simulink model "VTOLAutopilotController"  (R2025a)
settings: configuration reference "VTOLConfiguration" (kept outside this file)
undefined symbols (not defined in the file): Back_Transition_Rate, const, control, controlParams, ControlSampleTime, CriticalTiltAngle, DiscIntNeverNeededParam, dspblkCoreblockFVToolHelper, Fading_time, flightState, FSState, FWControlParams, FWTrimSpeed, gcbh, HoverMission, ReferenceFilterDen, ReferenceFilterNum, tilt_max, tiltIni, TransitioncontrolGains, uavParam, uavParams, VTOLcontrolGains, w_trim, WindDownRate
libraries: simulink x43, slpidlib x35, uavalgslib x7, simulink_extras x1
(part 5 of 8)

== system VTOLAutopilotController/Low level controller/Fixed Wing Controller/Fixed Wing Controller Module/Fixed Wing Controller Tuning/Airspeed-Altitude Controller ==
  note: Airspeed and altitude are controlled independently
      | by ignoring their coupled dynamics.
  Airspeed SP : Inport
  Altitude SP : Inport  Port=2
  Climb Rate SP : Inport  Port=3
  Airspeed : Inport  Port=4
  xyz : Inport  Port=5
  vxyz : Inport  Port=6
  Enable : EnablePort  ShowOutputPort=on
  Airspeed Controller : slpidlib/PID Controller  Controller=PID  Form=Parallel  TimeDomain=Discrete-time  UseExternalTs=off  SampleTime=ControlSampleTime  IntegratorMethod=Trapezoidal  FilterMethod=Forward Euler  ControllerParametersSource=internal  P=40.1166410885074  I=21.6851560041072  UseKiTs=off  D=2.18528545905044  UseExternalDerivativeSource=off  N=172.44752694034  UseFilter=on  TunerSelectOption=Transfer Function Based (PID Tuner App)  InitialConditionSource=internal  InitialConditionForIntegrator=0  InitialConditionForFilter=0  DifferentiatorICPrevScaledInput=0  ExternalReset=none  TrackingMode=off  Kt=1  LimitOutput=off  SatLimitsSource=internal  UpperSaturationLimit=Inf  LowerSaturationLimit=0  LinearizeAsGain=on  AntiWindupMode=clamping  Kb=1  LimitIntegrator=off  UpperIntegratorSaturationLimit=inf  LowerIntegratorSaturationLimit=-inf  POutMin=[]  POutMax=[]  IOutMin=[]  IOutMax=[]  DOutMin=[]  DOutMax=[]  NOutMin=[]  NOutMax=[]  SumOutMin=[]  SumOutMax=[]  SaturationOutMin=[]  SaturationOutMax=[]  PParamMin=[]  PParamMax=[]  IParamMin=[]  IParamMax=[]  DParamMin=[]  DParamMax=[]  NParamMin=[]  NParamMax=[]  KbParamMin=[]  KbParamMax=[]  KtParamMin=[]  KtParamMax=[]  KbOutMin=[]  KbOutMax=[]  KtOutMin=[]  KtOutMax=[]  IntegratorOutMin=[]  IntegratorOutMax=[]  FilterOutMin=[]  FilterOutMax=[]  SumI1OutMin=[]  SumI1OutMax=[]  SumI2OutMin=[]  SumI2OutMax=[]  SumI3OutMin=[]  SumI3OutMax=[]  SumI4OutMin=[]  SumI4OutMax=[]  SumDOutMin=[]  SumDOutMax=[]  DifferentiatorOutMin=[]  DifferentiatorOutMax=[]  FilterDiffOutCoefMin=[]  FilterDiffOutCoefMax=[]  ReciprocalOutMin=[]  ReciprocalOutMax=[]  SumDenOutMin=[]  SumDenOutMax=[]  SumNumOutMin=[]  SumNumOutMax=[]  DivideOutMin=[]  DivideOutMax=[]  UdiffTsProdOutMin=[]  UdiffTsProdOutMax=[]  NTsProdOutMin=[]  NTsProdOutMax=[]  UintegralTsProdOutMin=[]  UintegralTsProdOutMax=[]  UngainTsProdOutMin=[]  UngainTsProdOutMax=[]  ClampingZeroOutDataTypeStr=Inherit: Inherit via back propagation  ClampingZeroOutMin=[]  ClampingZeroOutMax=[]  FilterDenConstantOutDataTypeStr=Inherit: Inherit via back propagation  FilterDenConstantOutMin=[]  FilterDenConstantOutMax=[]  PCopyOutDataTypeStr=Inherit: Inherit via back propagation  PCopyOutMin=[]  PCopyOutMax=[]  NCopyOutDataTypeStr=Inherit: Inherit via back propagation  NCopyOutMin=[]  NCopyOutMax=[]  IntegratorContinuousStateAttributes=''  IntegratorStateMustResolveToSignalObject=off  IntegratorRTWStateStorageClass=Auto  FilterContinuousStateAttributes=''  FilterStateMustResolveToSignalObject=off  FilterRTWStateStorageClass=Auto  ParallelPVariant=InternalParameters  IdealPVariant=Disabled  IVariant=InternalParameters  DVariant=InternalParameters  IntegratorVariant=Discrete  SatVariant=Disabled  AWVariant=Passthrough  PCopyVariant=Disabled  TRVariant=Disabled  FdbkBlocksVariant=Forward  IdealPFdbkVariant=Disabled  SatFdbkVariant=Disabled  DerivativeFilterVariant=ForwardEulerFilter  NVariant=InternalParameters  NCopyVariant=Disabled  FilterICVariant=InternalICsFilter  IntegratorICVariant=InternalICs  ExternalResetVariant=Disabled  TRSumVariant=Passthrough  SumFdbkVariant=Disabled  SumVariant=Sum_PID  TsampFilterVariant=InternalTs  TsampNgainVariant=Passthrough  TsampIntegralVariant=Disabled_SignalSpec  ExternalSaturationOutDataTypeStr=Inherit: Same as second input  DerivativeSourceVariant=ErrorSignal  PreIntVariant=InternalPreInt
  Altitude Controller : Subsystem
  Climb Rate SP Switch : Switch  Criteria=u2 > Threshold  SaturateOnIntegerOverflow=off  InputSameDT=off
  Climb Rate SP from Guidance : Subsystem  TreatAsAtomicUnit=on
  Compare To Constant : simulink/Logic and Bit Operations/Compare To Constant  relop===  const=uint8(1)  OutDataTypeStr=boolean
  Compare To Constant1 : simulink/Logic and Bit Operations/Compare To Constant  relop===  const=uint8(2)  OutDataTypeStr=boolean
  Pitch SP Controller : Subsystem
  Sum1 : Sum  Inputs=|+-
  Pitch SP : Outport
  Throttle : Outport  Port=2
  wires:
  Airspeed SP/1 -> Sum1/1
  Sum1/1 -> Airspeed Controller/1
  Airspeed/1 -> Sum1/2
  Airspeed Controller/1 -> Throttle/1
  Altitude SP/1 -> Altitude Controller/1(Alt SP)
  xyz/1 -> Altitude Controller/2(xyz)
  vxyz/1 -> Pitch SP Controller/2(vxyz)
  Pitch SP Controller/1(Pitch SP) -> Pitch SP/1
  Enable/1 -> Compare To Constant1/1, Compare To Constant/1
  Compare To Constant/1 -> Climb Rate SP Switch/2, Altitude Controller/Enable
  Compare To Constant1/1 -> Climb Rate SP from Guidance/Enable
  Altitude Controller/1(Climb Rate SP) -> Climb Rate SP Switch/1
  Climb Rate SP from Guidance/1(Out1) -> Climb Rate SP Switch/3
  Climb Rate SP Switch/1 -> Pitch SP Controller/1(Climb Rate SP)
  Climb Rate SP/1 -> Climb Rate SP from Guidance/1(Climb Rate SP)

== system VTOLAutopilotController/Low level controller/Fixed Wing Controller/Fixed Wing Controller Module/Fixed Wing Controller Tuning/Attitude Controller ==
  YPR SP : Inport
  ypr : Inport  Port=2
  Ang Rate : Inport  Port=3
  Airspeed : Inport  Port=4
  Enable : EnablePort  ShowOutputPort=on
  AER Switch : Switch  Criteria=u2 > Threshold  SaturateOnIntegerOverflow=off  InputSameDT=off
  Compare To Constant : simulink/Logic and Bit Operations/Compare To Constant  relop===  const=uint8(1)  OutDataTypeStr=boolean
  Compare To Constant1 : simulink/Logic and Bit Operations/Compare To Constant  relop===  const=uint8(2)  OutDataTypeStr=boolean
  Demux1 : Demux  Outputs=3
  Pitch Roll Controller : Subsystem
  Rudder Heading Controller : Subsystem
  AER : Outport
  wires:
  ypr/1 -> Rudder Heading Controller/2(YPR), Pitch Roll Controller/3(YPR)
  YPR SP/1 -> Demux1/1
  Enable/1 -> Compare To Constant1/1, Compare To Constant/1
  AER Switch/1 -> AER/1
  Compare To Constant/1 -> AER Switch/2, Pitch Roll Controller/Enable
  Pitch Roll Controller/1(AER) -> AER Switch/1
  Rudder Heading Controller/1(AER) -> AER Switch/3
  Demux1/1 -> Rudder Heading Controller/1(Yaw SP)
  Demux1/2 -> Pitch Roll Controller/1(Pitch SP)
  Demux1/3 -> Pitch Roll Controller/2(Roll SP)
  Ang Rate/1 -> Rudder Heading Controller/3(Ang Rate), Pitch Roll Controller/4(Ang Rate)
  Compare To Constant1/1 -> Rudder Heading Controller/Enable
  Airspeed/1 -> Pitch Roll Controller/5(Airspeed)

== system VTOLAutopilotController/Low level controller/Fixed Wing Controller/Fixed Wing Controller Module/Fixed Wing Controller Tuning/Lateral Guidance Logic ==
  note: S. Park, J. Deyst, and J. P. How, "A New Nonlinear Guidance Logic for Trajectory Tracking," Proceedings of the AIAA Guidance, Navigation and Control Conference, Aug 2004. AIAA-2004-4900.
  Course SP : Inport
  L1 Distance : Inport  Port=2
  course : Inport  Port=3
  gndspeed : Inport  Port=4
  Enable : EnablePort
  MATLAB Function : MATLAB Function  TreatAsAtomicUnit=on  SystemSampleTime=ControlSampleTime
  Terminator : Terminator
  Roll SP : Outport
  wires:
  Course SP/1 -> MATLAB Function/1(courseSP)
  course/1 -> MATLAB Function/2(course)
  MATLAB Function/2(rollSP) -> Roll SP/1
  MATLAB Function/1(lacc) -> Terminator/1
  gndspeed/1 -> MATLAB Function/3(groundSpeed)
  L1 Distance/1 -> MATLAB Function/4(L1)

== system VTOLAutopilotController/Low level controller/Fixed Wing Controller/Fixed Wing Controller Module/Fixed Wing Controller Tuning/Pitch, Airspeed SP from Controller ==
  Pitch SP In : Inport
  Airspeed SP : Inport  Port=2
  Airspeed : Inport  Port=3
  Enable : EnablePort
  Airspeed Controller : slpidlib/PID Controller  Controller=PID  Form=Parallel  TimeDomain=Discrete-time  UseExternalTs=off  SampleTime=ControlSampleTime  IntegratorMethod=Trapezoidal  FilterMethod=Forward Euler  ControllerParametersSource=internal  P=FWControlParams.P_AIRSPD  I=FWControlParams.I_AIRSPD  UseKiTs=off  D=FWControlParams.D_AIRSPD  UseExternalDerivativeSource=off  N=FWControlParams.N_AIRSPD  UseFilter=on  TunerSelectOption=Transfer Function Based (PID Tuner App)  InitialConditionSource=internal  InitialConditionForIntegrator=0  InitialConditionForFilter=0  DifferentiatorICPrevScaledInput=0  ExternalReset=none  TrackingMode=off  Kt=1  LimitOutput=off  SatLimitsSource=internal  UpperSaturationLimit=Inf  LowerSaturationLimit=0  LinearizeAsGain=on  AntiWindupMode=clamping  Kb=1  LimitIntegrator=off  UpperIntegratorSaturationLimit=inf  LowerIntegratorSaturationLimit=-inf  POutMin=[]  POutMax=[]  IOutMin=[]  IOutMax=[]  DOutMin=[]  DOutMax=[]  NOutMin=[]  NOutMax=[]  SumOutMin=[]  SumOutMax=[]  SaturationOutMin=[]  SaturationOutMax=[]  PParamMin=[]  PParamMax=[]  IParamMin=[]  IParamMax=[]  DParamMin=[]  DParamMax=[]  NParamMin=[]  NParamMax=[]  KbParamMin=[]  KbParamMax=[]  KtParamMin=[]  KtParamMax=[]  KbOutMin=[]  KbOutMax=[]  KtOutMin=[]  KtOutMax=[]  IntegratorOutMin=[]  IntegratorOutMax=[]  FilterOutMin=[]  FilterOutMax=[]  SumI1OutMin=[]  SumI1OutMax=[]  SumI2OutMin=[]  SumI2OutMax=[]  SumI3OutMin=[]  SumI3OutMax=[]  SumI4OutMin=[]  SumI4OutMax=[]  SumDOutMin=[]  SumDOutMax=[]  DifferentiatorOutMin=[]  DifferentiatorOutMax=[]  FilterDiffOutCoefMin=[]  FilterDiffOutCoefMax=[]  ReciprocalOutMin=[]  ReciprocalOutMax=[]  SumDenOutMin=[]  SumDenOutMax=[]  SumNumOutMin=[]  SumNumOutMax=[]  DivideOutMin=[]  DivideOutMax=[]  UdiffTsProdOutMin=[]  UdiffTsProdOutMax=[]  NTsProdOutMin=[]  NTsProdOutMax=[]  UintegralTsProdOutMin=[]  UintegralTsProdOutMax=[]  UngainTsProdOutMin=[]  UngainTsProdOutMax=[]  ClampingZeroOutDataTypeStr=Inherit: Inherit via back propagation  ClampingZeroOutMin=[]  ClampingZeroOutMax=[]  FilterDenConstantOutDataTypeStr=Inherit: Inherit via back propagation  FilterDenConstantOutMin=[]  FilterDenConstantOutMax=[]  PCopyOutDataTypeStr=Inherit: Inherit via back propagation  PCopyOutMin=[]  PCopyOutMax=[]  NCopyOutDataTypeStr=Inherit: Inherit via back propagation  NCopyOutMin=[]  NCopyOutMax=[]  IntegratorContinuousStateAttributes=''  IntegratorStateMustResolveToSignalObject=off  IntegratorRTWStateStorageClass=Auto  FilterContinuousStateAttributes=''  FilterStateMustResolveToSignalObject=off  FilterRTWStateStorageClass=Auto  ParallelPVariant=InternalParameters  IdealPVariant=Disabled  IVariant=InternalParameters  DVariant=InternalParameters  IntegratorVariant=Discrete  SatVariant=Disabled  AWVariant=Passthrough  PCopyVariant=Disabled  TRVariant=Disabled  FdbkBlocksVariant=Forward  IdealPFdbkVariant=Disabled  SatFdbkVariant=Disabled  DerivativeFilterVariant=ForwardEulerFilter  NVariant=InternalParameters  NCopyVariant=Disabled  FilterICVariant=InternalICsFilter  IntegratorICVariant=InternalICs  ExternalResetVariant=Disabled  TRSumVariant=Passthrough  SumFdbkVariant=Disabled  SumVariant=Sum_PID  TsampFilterVariant=InternalTs  TsampNgainVariant=Passthrough  TsampIntegralVariant=Disabled_SignalSpec  ExternalSaturationOutDataTypeStr=Inherit: Same as second input  DerivativeSourceVariant=ErrorSignal  PreIntVariant=InternalPreInt
  IC : InitialCondition  Value=0
  Sum1 : Sum  Inputs=|+-
  Pitch SP : Outport
  Throttle : Outport  Port=2
  wires:
  IC/1 -> Pitch SP/1
  Pitch SP In/1 -> IC/1
  Airspeed SP/1 -> Sum1/1
  Sum1/1 -> Airspeed Controller/1
  Airspeed/1 -> Sum1/2
  Airspeed Controller/1 -> Throttle/1

== system VTOLAutopilotController/Low level controller/Fixed Wing Controller/Fixed Wing Controller Module/Fixed Wing Controller Tuning/Roll SP from Path Manager ==
  In1 : Inport
  Enable : EnablePort
  IC : InitialCondition  Value=0
  Out1 : Outport
  wires:
  In1/1 -> IC/1
  IC/1 -> Out1/1

== system VTOLAutopilotController/Low level controller/Fixed Wing Controller/Fixed Wing Controller Module/Fixed Wing Controller Tuning/Subsystem2 ==
  Euler : Inport
  pqr : Inport  Port=2
  Demux : Demux  Outputs=3
  Display : Display
  MATLAB Function : MATLAB Function  TreatAsAtomicUnit=on
  Matrix Multiply : Product  Multiplication=Matrix(*)
  Terminator : Terminator
  Euler Rate : Outport
  wires:
  Demux/1 -> MATLAB Function/1(phi)
  Demux/2 -> MATLAB Function/2(theta)
  MATLAB Function/1(y) -> Matrix Multiply/1
  pqr/1 -> Matrix Multiply/2
  Euler/1 -> Demux/1
  Demux/3 -> Terminator/1
  Matrix Multiply/1 -> Display/1, Euler Rate/1

== system VTOLAutopilotController/Low level controller/Multicopter Controller/Attitude & Altitude controller/Altitude Control/Alt signal condition ==
  Z_in : Inport
  Constant : Constant  Value=0  SampleTime=-1
  Gain : Gain  Gain=-1
  Gain1 : Gain  Gain=-1
  Saturation Dynamic : simulink/Discontinuities/Saturation Dynamic  OutMin=[]  OutMax=[]  OutDataTypeStr=Inherit: Same as second input  OutDataType=fixdt(1, 16)  OutScaling=2^-10  DoSatur=off
  Z_out : Outport
  wires:
  Z_in/1 -> Gain/1
  Gain/1 -> Saturation Dynamic/1, Saturation Dynamic/2
  Constant/1 -> Saturation Dynamic/3
  Saturation Dynamic/1 -> Gain1/1
  Gain1/1 -> Z_out/1

== system VTOLAutopilotController/Low level controller/Multicopter Controller/Attitude & Altitude controller/Altitude Control/Triggered Subsystem ==
  AltHold : Inport
  Trigger : TriggerPort  VariantControl=(inherit)
  Reference : Outport
  wires:
  AltHold/1 -> Reference/1

== system VTOLAutopilotController/Low level controller/Multicopter Controller/Horizontal Position Control/XY Controller/Forward position ==
  e_y : Inport
  e_x : Inport  Port=2
  sin : Inport  Port=3
  cos : Inport  Port=4
  Add : Sum
  Product : Product
  Product1 : Product
  ef : Outport
  wires:
  Add/1 -> ef/1
  Product1/1 -> Add/2
  Product/1 -> Add/1
  e_x/1 -> Product/2
  e_y/1 -> Product1/1
  sin/1 -> Product1/2
  cos/1 -> Product/1

== system VTOLAutopilotController/Low level controller/Multicopter Controller/Horizontal Position Control/XY Controller/Forward velocity ==
  vy : Inport
  vx : Inport  Port=2
  sin : Inport  Port=3
  cos : Inport  Port=4
  Add : Sum
  Product : Product
  Product1 : Product
  ef : Outport
  wires:
  cos/1 -> Product/1
  sin/1 -> Product1/2
  vy/1 -> Product1/1
  vx/1 -> Product/2
  Product/1 -> Add/1
  Product1/1 -> Add/2
  Add/1 -> ef/1

== system VTOLAutopilotController/Low level controller/Multicopter Controller/Horizontal Position Control/XY Controller/Lateral position ==
  e_y : Inport
  e_x : Inport  Port=2
  sin : Inport  Port=3
  cos : Inport  Port=4
  Add : Sum
  Gain : Gain  Gain=-1
  Product : Product
  Product1 : Product
  el : Outport
  wires:
  e_y/1 -> Product1/1
  e_x/1 -> Product/2
  sin/1 -> Product/1
  cos/1 -> Product1/2
  Product/1 -> Gain/1
  Product1/1 -> Add/2
  Add/1 -> el/1
  Gain/1 -> Add/1

== system VTOLAutopilotController/Low level controller/Multicopter Controller/Horizontal Position Control/XY Controller/Lateral velocity ==
  vy : Inport
  vx : Inport  Port=2
  sin : Inport  Port=3
  cos : Inport  Port=4
  Add : Sum
  Gain : Gain  Gain=-1
  Product : Product
  Product1 : Product
  el : Outport
  wires:
  Gain/1 -> Add/1
  Add/1 -> el/1
  Product1/1 -> Add/2
  Product/1 -> Gain/1
  cos/1 -> Product1/2
  sin/1 -> Product/1
  vx/1 -> Product/2
  vy/1 -> Product1/1

== system VTOLAutopilotController/Low level controller/Scheduler/FixedWingScheduler/Switch Case Action Subsystem3/Signal_Fader_OnOff1 ==
  SW : Inport
  Input_On : Inport  Port=2
  Input_Off : Inport  Port=3
  Fading_Time : Inport  Port=4
  Compare To Constant : simulink/Logic and Bit Operations/Compare To Constant  relop===  const=0  OutDataTypeStr=boolean
  Fader_Off : Subsystem
  Fader_On : Subsystem
  Product : Product
  Product1 : Product
  Sum{,1..3} (4 alike) : Sum  Inputs=+-
  Switch : Switch  Criteria=u2 > Threshold  SaturateOnIntegerOverflow=off  InputSameDT=off
  Switch1 : Switch  Criteria=u2 > Threshold  SaturateOnIntegerOverflow=off  InputSameDT=off
  Switch2 : Switch  Criteria=u2 > Threshold  SaturateOnIntegerOverflow=off  InputSameDT=off
  Unit Delay : UnitDelay  SampleTime=-1  HasFrameUpgradeWarning=on
  Unit Delay1 : UnitDelay  SampleTime=-1  HasFrameUpgradeWarning=on
  Unit Delay2 : UnitDelay  SampleTime=-1  HasFrameUpgradeWarning=on
  Out : Outport
  wires:
  SW/1 -> [Engage]
  Fading_Time/1 -> [Fade_Time]
  [Engage] -> Fader_On/1(SW)
  [Fade_Time] -> Fader_On/2(Fader_Time)
  [Engage] -> Compare To Constant/1
  Compare To Constant/1 -> Fader_Off/1(SW)
  [Fade_Time] -> Fader_Off/2(Fader_Time)
  Input_On/1 -> [On_Input]
  Input_Off/1 -> [Off_Input]
  Unit Delay/1 -> [Out_Capture]
  Switch/1 -> Unit Delay/1, Out/1
  [On_Input] -> Sum/1
  Sum/1 -> Switch/1
  [On_Input] -> Sum1/1
  [Out_Capture] -> Sum1/2
  Sum1/1 -> Switch1/3
  Switch1/1 -> Unit Delay1/1, Product/1
  Unit Delay1/1 -> Switch1/1
  [Engage] -> Switch1/2
  Product/1 -> Sum/2
  Fader_On/1(On) -> Product/2
  [Engage] -> Switch/2
  Sum2/1 -> Switch/3
  Product1/1 -> Sum2/2
  [Off_Input] -> Sum2/1
  [Off_Input] -> Sum3/1
  [Engage] -> Switch2/2
  [Out_Capture] -> Sum3/2
  Sum3/1 -> Switch2/1
  Switch2/1 -> Unit Delay2/1, Product1/2
  Unit Delay2/1 -> Switch2/3
  Fader_Off/1(On) -> Product1/1

== system VTOLAutopilotController/Low level controller/Scheduler/Subsystem/Switch Case Action Subsystem3/Signal_Fader_OnOff ==
  SW : Inport
  Input_On : Inport  Port=2
  Input_Off : Inport  Port=3
  Fading_Time : Inport  Port=4
  Compare To Constant : simulink/Logic and Bit Operations/Compare To Constant  relop===  const=0  OutDataTypeStr=boolean
  Fader_Off : Subsystem
  Fader_On : Subsystem
  Product : Product
  Product1 : Product
  Sum{,1..3} (4 alike) : Sum  Inputs=+-
  Switch : Switch  Criteria=u2 > Threshold  SaturateOnIntegerOverflow=off  InputSameDT=off
  Switch1 : Switch  Criteria=u2 > Threshold  SaturateOnIntegerOverflow=off  InputSameDT=off
  Switch2 : Switch  Criteria=u2 > Threshold  SaturateOnIntegerOverflow=off  InputSameDT=off
  Unit Delay : UnitDelay  SampleTime=-1  HasFrameUpgradeWarning=on
  Unit Delay1 : UnitDelay  SampleTime=-1  HasFrameUpgradeWarning=on
  Unit Delay2 : UnitDelay  SampleTime=-1  HasFrameUpgradeWarning=on
  Out : Outport
  wires:
  SW/1 -> [Engage]
  Fading_Time/1 -> [Fade_Time]
  [Engage] -> Fader_On/1(SW)
  [Fade_Time] -> Fader_On/2(Fader_Time)
  [Engage] -> Compare To Constant/1
  Compare To Constant/1 -> Fader_Off/1(SW)
  [Fade_Time] -> Fader_Off/2(Fader_Time)
  Input_On/1 -> [On_Input]
  Input_Off/1 -> [Off_Input]
  Unit Delay/1 -> [Out_Capture]
  Switch/1 -> Unit Delay/1, Out/1
  [On_Input] -> Sum/1
  Sum/1 -> Switch/1
  [On_Input] -> Sum1/1
  [Out_Capture] -> Sum1/2
  Sum1/1 -> Switch1/3
  Switch1/1 -> Unit Delay1/1, Product/1
  Unit Delay1/1 -> Switch1/1
  [Engage] -> Switch1/2
  Product/1 -> Sum/2
  Fader_On/1(On) -> Product/2
  [Engage] -> Switch/2
  Sum2/1 -> Switch/3
  Product1/1 -> Sum2/2
  [Off_Input] -> Sum2/1
  [Off_Input] -> Sum3/1
  [Engage] -> Switch2/2
  [Out_Capture] -> Sum3/2
  Sum3/1 -> Switch2/1
  Switch2/1 -> Unit Delay2/1, Product1/2
  Unit Delay2/1 -> Switch2/3
  Fader_Off/1(On) -> Product1/1

== system VTOLAutopilotController/Low level controller/Scheduler/Subsystem/Switch Case Action Subsystem3/Signal_Fader_OnOff1 ==
  SW : Inport
  Input_On : Inport  Port=2
  Input_Off : Inport  Port=3
  Fading_Time : Inport  Port=4
  Compare To Constant : simulink/Logic and Bit Operations/Compare To Constant  relop===  const=0  OutDataTypeStr=boolean
  Fader_Off : Subsystem
  Fader_On : Subsystem
  Product : Product
  Product1 : Product
  Sum{,1..3} (4 alike) : Sum  Inputs=+-
  Switch : Switch  Criteria=u2 > Threshold  SaturateOnIntegerOverflow=off  InputSameDT=off
  Switch1 : Switch  Criteria=u2 > Threshold  SaturateOnIntegerOverflow=off  InputSameDT=off
  Switch2 : Switch  Criteria=u2 > Threshold  SaturateOnIntegerOverflow=off  InputSameDT=off
  Unit Delay : UnitDelay  SampleTime=-1  HasFrameUpgradeWarning=on
  Unit Delay1 : UnitDelay  SampleTime=-1  HasFrameUpgradeWarning=on
  Unit Delay2 : UnitDelay  SampleTime=-1  HasFrameUpgradeWarning=on
  Out : Outport
  wires:
  SW/1 -> [Engage]
  Fading_Time/1 -> [Fade_Time]
  [Engage] -> Fader_On/1(SW)
  [Fade_Time] -> Fader_On/2(Fader_Time)
  [Engage] -> Compare To Constant/1
  Compare To Constant/1 -> Fader_Off/1(SW)
  [Fade_Time] -> Fader_Off/2(Fader_Time)
  Input_On/1 -> [On_Input]
  Input_Off/1 -> [Off_Input]
  Unit Delay/1 -> [Out_Capture]
  Switch/1 -> Unit Delay/1, Out/1
  [On_Input] -> Sum/1
  Sum/1 -> Switch/1
  [On_Input] -> Sum1/1
  [Out_Capture] -> Sum1/2
  Sum1/1 -> Switch1/3
  Switch1/1 -> Unit Delay1/1, Product/1
  Unit Delay1/1 -> Switch1/1
  [Engage] -> Switch1/2
  Product/1 -> Sum/2
  Fader_On/1(On) -> Product/2
  [Engage] -> Switch/2
  Sum2/1 -> Switch/3
  Product1/1 -> Sum2/2
  [Off_Input] -> Sum2/1
  [Off_Input] -> Sum3/1
  [Engage] -> Switch2/2
  [Out_Capture] -> Sum3/2
  Sum3/1 -> Switch2/1
  Switch2/1 -> Unit Delay2/1, Product1/2
  Unit Delay2/1 -> Switch2/3
  Fader_Off/1(On) -> Product1/1

== system VTOLAutopilotController/Low level controller/Scheduler/Subsystem/Switch Case Action Subsystem3/Signal_Fader_OnOff2 ==
  SW : Inport
  Input_On : Inport  Port=2
  Input_Off : Inport  Port=3
  Fading_Time : Inport  Port=4
  Compare To Constant : simulink/Logic and Bit Operations/Compare To Constant  relop===  const=0  OutDataTypeStr=boolean
  Fader_Off : Subsystem
  Fader_On : Subsystem
  Product : Product
  Product1 : Product
  Sum{,1..3} (4 alike) : Sum  Inputs=+-
  Switch : Switch  Criteria=u2 > Threshold  SaturateOnIntegerOverflow=off  InputSameDT=off
  Switch1 : Switch  Criteria=u2 > Threshold  SaturateOnIntegerOverflow=off  InputSameDT=off
  Switch2 : Switch  Criteria=u2 > Threshold  SaturateOnIntegerOverflow=off  InputSameDT=off
  Unit Delay : UnitDelay  SampleTime=-1  HasFrameUpgradeWarning=on
  Unit Delay1 : UnitDelay  SampleTime=-1  HasFrameUpgradeWarning=on
  Unit Delay2 : UnitDelay  SampleTime=-1  HasFrameUpgradeWarning=on
  Out : Outport
  wires:
  SW/1 -> [Engage]
  Fading_Time/1 -> [Fade_Time]
  [Engage] -> Fader_On/1(SW)
  [Fade_Time] -> Fader_On/2(Fader_Time)
  [Engage] -> Compare To Constant/1
  Compare To Constant/1 -> Fader_Off/1(SW)
  [Fade_Time] -> Fader_Off/2(Fader_Time)
  Input_On/1 -> [On_Input]
  Input_Off/1 -> [Off_Input]
  Unit Delay/1 -> [Out_Capture]
  Switch/1 -> Unit Delay/1, Out/1
  [On_Input] -> Sum/1
  Sum/1 -> Switch/1
  [On_Input] -> Sum1/1
  [Out_Capture] -> Sum1/2
  Sum1/1 -> Switch1/3
  Switch1/1 -> Unit Delay1/1, Product/1
  Unit Delay1/1 -> Switch1/1
  [Engage] -> Switch1/2
  Product/1 -> Sum/2
  Fader_On/1(On) -> Product/2
  [Engage] -> Switch/2
  Sum2/1 -> Switch/3
  Product1/1 -> Sum2/2
  [Off_Input] -> Sum2/1
  [Off_Input] -> Sum3/1
  [Engage] -> Switch2/2
  [Out_Capture] -> Sum3/2
  Sum3/1 -> Switch2/1
  Switch2/1 -> Unit Delay2/1, Product1/2
  Unit Delay2/1 -> Switch2/3
  Fader_Off/1(On) -> Product1/1

== system VTOLAutopilotController/Low level controller/Scheduler/Subsystem/Switch Case Action Subsystem3/Signal_Fader_OnOff3 ==
  SW : Inport
  Input_On : Inport  Port=2
  Input_Off : Inport  Port=3
  Fading_Time : Inport  Port=4
  Compare To Constant : simulink/Logic and Bit Operations/Compare To Constant  relop===  const=0  OutDataTypeStr=boolean
  Fader_Off : Subsystem
  Fader_On : Subsystem
  Product : Product
  Product1 : Product
  Sum{,1..3} (4 alike) : Sum  Inputs=+-
  Switch : Switch  Criteria=u2 > Threshold  SaturateOnIntegerOverflow=off  InputSameDT=off
  Switch1 : Switch  Criteria=u2 > Threshold  SaturateOnIntegerOverflow=off  InputSameDT=off
  Switch2 : Switch  Criteria=u2 > Threshold  SaturateOnIntegerOverflow=off  InputSameDT=off
  Unit Delay : UnitDelay  SampleTime=-1  HasFrameUpgradeWarning=on
  Unit Delay1 : UnitDelay  SampleTime=-1  HasFrameUpgradeWarning=on
  Unit Delay2 : UnitDelay  SampleTime=-1  HasFrameUpgradeWarning=on
  Out : Outport
  wires:
  SW/1 -> [Engage]
  Fading_Time/1 -> [Fade_Time]
  [Engage] -> Fader_On/1(SW)
  [Fade_Time] -> Fader_On/2(Fader_Time)
  [Engage] -> Compare To Constant/1
  Compare To Constant/1 -> Fader_Off/1(SW)
  [Fade_Time] -> Fader_Off/2(Fader_Time)
  Input_On/1 -> [On_Input]
  Input_Off/1 -> [Off_Input]
  Unit Delay/1 -> [Out_Capture]
  Switch/1 -> Unit Delay/1, Out/1
  [On_Input] -> Sum/1
  Sum/1 -> Switch/1
  [On_Input] -> Sum1/1
  [Out_Capture] -> Sum1/2
  Sum1/1 -> Switch1/3
  Switch1/1 -> Unit Delay1/1, Product/1
  Unit Delay1/1 -> Switch1/1
  [Engage] -> Switch1/2
  Product/1 -> Sum/2
  Fader_On/1(On) -> Product/2
  [Engage] -> Switch/2
  Sum2/1 -> Switch/3
  Product1/1 -> Sum2/2
  [Off_Input] -> Sum2/1
  [Off_Input] -> Sum3/1
  [Engage] -> Switch2/2
  [Out_Capture] -> Sum3/2
  Sum3/1 -> Switch2/1
  Switch2/1 -> Unit Delay2/1, Product1/2
  Unit Delay2/1 -> Switch2/3
  Fader_Off/1(On) -> Product1/1

== system VTOLAutopilotController/Guidance Test Bench/ControlType/Guidance Testbench/Guidance Logic/Guidance Stateflow/Guidance Mode Selector/GuidanceLogic.BackTransition.BackTransition ==
  note: Flight Mode Manager
  States : Inport
  Action Port : ActionPort
      settings: CopyFcn=Stateflow.SLINSF.SimulinkMan.removeBlockPreDeleteFcn  PreDeleteFcn=Stateflow.SLINSF.SimulinkMan.unsafePredeleteFcn
  Bus Creator1 : BusCreator  Inputs=2  OutDataTypeStr=Bus: LAPY  NonVirtualBus=on
  Bus Selector : BusSelector  OutputSignals=Xe
  Bus Selector1 : BusSelector  OutputSignals=Ve,Tilt
  Constant1 : Constant  Value=0
  Constant2 : Constant  Value=0
  Data Type Conversion : DataTypeConversion  OutDataTypeStr=uint8  SaturateOnIntegerOverflow=off  RndMeth=Floor
  Gain : Gain
  MATLAB Function : MATLAB Function  TreatAsAtomicUnit=on
  Terminator : Terminator
  Terminator1 : Terminator
  Status : Outport
  wires:
  Bus Selector1/1 -> MATLAB Function/1(Vb)  "<Ve>"
  States/1 -> Bus Selector/1, Bus Selector1/1
  Bus Selector/1 -> Gain/1  "<Xe>"
  Bus Creator1/1 -> Terminator1/1
  Constant2/1 -> Bus Creator1/2  "yaw"
  MATLAB Function/1(flag) -> Data Type Conversion/1
  Data Type Conversion/1 -> Status/1
  Bus Selector1/2 -> MATLAB Function/2(tilt)  "<Tilt>"
  Gain/1 -> Bus Creator1/1  "localposition"
  Constant1/1 -> Terminator/1  "HeadingCmd"

== system VTOLAutopilotController/Guidance Test Bench/ControlType/Guidance Testbench/Guidance Logic/Guidance Stateflow/Guidance Mode Selector/GuidanceLogic.FIXED_WING_ORBIT.ORBIT ==
  ToWP : Inport
  States : Inport  Port=2
  Action Port : ActionPort
      settings: CopyFcn=Stateflow.SLINSF.SimulinkMan.removeBlockPreDeleteFcn  PreDeleteFcn=Stateflow.SLINSF.SimulinkMan.unsafePredeleteFcn
  Abs1 : Abs  SaturateOnIntegerOverflow=off
  Bus Creator : BusCreator  Inputs=5  OutDataTypeStr=Bus: AAC  NonVirtualBus=on
      settings: InheritFromInputs=off
  Bus Selector : BusSelector  OutputSignals=position,params
  Bus Selector1 : BusSelector  OutputSignals=Xe,course  OutputAsBus=on
  Bus to Vector : BusToVector
  Constant : Constant  Value=control.cruiseSpeed
  Constant1 : Constant  Value=0
  Data Type Conversion : DataTypeConversion  OutDataTypeStr=uint8  SaturateOnIntegerOverflow=off  RndMeth=Floor
  Lookahead Distance : Constant  Value=control.L1  OutDataTypeStr=double
  Relational Operator : RelationalOperator  Operator=>  OutDataTypeStr=boolean  RndMeth=Simplest  InputSameDT=off
  Selector : Selector  InputPortWidth=3  IndexOptions=Index vector (dialog)  Indices=3  OutputSizes=1
  Selector1 : Selector  InputPortWidth=4  IndexOptions=Index vector (dialog)  Indices=2  OutputSizes=1
  Selector2 : Selector  InputPortWidth=4  IndexOptions=Index vector (dialog)  Indices=1  OutputSizes=1
  Selector3 : Selector  InputPortWidth=4  IndexOptions=Index vector (dialog)  Indices=3  OutputSizes=1
  Terminator{,1..3} (4 alike) : Terminator
  UAV Orbit Follower : uavalgslib/Orbit Follower  UAVType=fixed-wing  MinOrbitRadius=control.turningRadius  MinLookaheadDistance=control.L1  ExternalReset=none  ShowCrossTrackErrorOutput=off  ShowNumTurnsOutput=on  SimulateUsing=Code generation
  Unary Minus : UnaryMinus
  Status : Outport
  AACSP : Outport  Port=2
  wires:
  Bus to Vector/1 -> UAV Orbit Follower/1
  Selector2/1 -> UAV Orbit Follower/3
  Bus Selector/1 -> UAV Orbit Follower/2, Selector/1  "<position>"
  ToWP/1 -> Bus Selector/1
  Bus Selector/2 -> Selector1/1, Selector3/1, Selector2/1  "<params>"
  Selector3/1 -> Relational Operator/2
  Relational Operator/1 -> Data Type Conversion/1
  UAV Orbit Follower/4 -> Terminator/1
  UAV Orbit Follower/5 -> Terminator1/1
  Bus Selector1/1 -> Bus to Vector/1
  States/1 -> Bus Selector1/1
  UAV Orbit Follower/1 -> Terminator2/1  "LAP"
  Lookahead Distance/1 -> UAV Orbit Follower/5, Bus Creator/4  "L1"
  Bus Creator/1 -> AACSP/1
  UAV Orbit Follower/2 -> Bus Creator/3  "course"
  Constant/1 -> Bus Creator/1  "airspeed"
  Unary Minus/1 -> Bus Creator/2  "altitude"
  UAV Orbit Follower/3 -> Terminator3/1  "YawCmd"
  Selector/1 -> Unary Minus/1
  UAV Orbit Follower/6 -> Abs1/1
  Abs1/1 -> Relational Operator/1
  Selector1/1 -> UAV Orbit Follower/4
  Constant1/1 -> Bus Creator/5  "climbrate"
  Data Type Conversion/1 -> Status/1

== system VTOLAutopilotController/Guidance Test Bench/ControlType/Guidance Testbench/Guidance Logic/Guidance Stateflow/Guidance Mode Selector/GuidanceLogic.FIXED_WING_WAYPOINT.WAYPOINT ==
  note: This subsystem selects a lookahead point on the path and provides a desired course. Desired course is later converted to desired lateral acceleration (and roll setpoint)
  States : Inport
  ToWP : Inport  Port=2
  FromWP : Inport  Port=3
  Action Port : ActionPort
      settings: CopyFcn=Stateflow.SLINSF.SimulinkMan.removeBlockPreDeleteFcn  PreDeleteFcn=Stateflow.SLINSF.SimulinkMan.unsafePredeleteFcn
  Bus Creator : BusCreator  Inputs=5  OutDataTypeStr=Bus: AAC  NonVirtualBus=on
      settings: InheritFromInputs=off
  Bus Selector : BusSelector  OutputSignals=Xe,course  OutputAsBus=on
  Bus Selector1 : BusSelector  OutputSignals=position
  Bus Selector2 : BusSelector  OutputSignals=position
  Bus Selector3 : BusSelector  OutputSignals=params
  Bus to Vector : BusToVector
  Constant1 : Constant  Value=0
  Constant3 : Constant  Value=controlParams.L1
  Data Type Conversion : DataTypeConversion  SaturateOnIntegerOverflow=off  RndMeth=Floor
  MATLAB Function : MATLAB Function  TreatAsAtomicUnit=on
  Selector : Selector  InputPortWidth=4  IndexOptions=Index vector (dialog)  Indices=[4]  OutputSizes=1
  Terminator : Terminator
  Terminator1 : Terminator
  Terminator2 : Terminator
  Waypoint Follower : uavalgslib/Waypoint Follower  UAVType=fixed-wing  StartFrom=first  TransitionRadiusSource=internal  TransitionRadius=FWControl.transitionRadius  MinLookaheadDistance=control.L1  HoverAtLastWaypoint=off  YawInput=off  ShowCrossTrackErrorOutput=off  ShowStatusOutput=on  SimulateUsing=Code generation
  Status : Outport
  AACSP : Outport  Port=2
  wires:
  Constant3/1 -> Waypoint Follower/3, Bus Creator/4  "L1"
  Waypoint Follower/1 -> Terminator/1  "LAP"
  Waypoint Follower/3 -> Terminator1/1  "YawCmd"
  Waypoint Follower/4 -> Terminator2/1
  States/1 -> Bus Selector/1
  Bus Selector/1 -> Bus to Vector/1
  Waypoint Follower/5 -> Data Type Conversion/1
  Data Type Conversion/1 -> Status/1
  Bus Creator/1 -> AACSP/1
  MATLAB Function/1(wps) -> Waypoint Follower/2
  Bus to Vector/1 -> Waypoint Follower/1
  ToWP/1 -> Bus Selector3/1, Bus Selector1/1
  FromWP/1 -> Bus Selector2/1
  Bus Selector1/1 -> MATLAB Function/1(toWP)  "<position>"
  Bus Selector2/1 -> MATLAB Function/2(fromWP)  "<position>"
  Constant1/1 -> Bus Creator/5  "climbrate"
  Bus Selector3/1 -> Selector/1  "<params>"
  Selector/1 -> Bus Creator/1  "airspeed"
  Waypoint Follower/2 -> [DesiredCourse]  "course"
  [DesiredCourse] -> Bus Creator/3  "course"
  MATLAB Function/2(alt) -> [AltCommand]  "alt"
  [AltCommand] -> Bus Creator/2  "alt"

== system VTOLAutopilotController/Guidance Test Bench/ControlType/Guidance Testbench/Guidance Logic/Guidance Stateflow/Guidance Mode Selector/GuidanceLogic.FixedWingEntry.FixedWingFlight.GuidanceInitialization ==
  States : Inport
  ToWP : Inport  Port=2
  FromWP : Inport  Port=3
  Action Port : ActionPort
      settings: CopyFcn=Stateflow.SLINSF.SimulinkMan.removeBlockPreDeleteFcn  PreDeleteFcn=Stateflow.SLINSF.SimulinkMan.unsafePredeleteFcn
  Bus Creator : BusCreator  Inputs=5  OutDataTypeStr=Bus: AAC  NonVirtualBus=on
      settings: InheritFromInputs=off
  Bus Selector2 : BusSelector  OutputSignals=position
  Bus Selector3 : BusSelector  OutputSignals=params
  Bus Selector4 : BusSelector  OutputSignals=Xe
  Constant1 : Constant  Value=0
  Constant3 : Constant  Value=controlParams.L1
  Constant4 : Constant  Value=0
  Constant5 : Constant  Value=0
  Data Type Conversion : DataTypeConversion  OutDataTypeStr=uint8  SaturateOnIntegerOverflow=off  RndMeth=Floor
  Gain : Gain  Gain=-1
  Selector : Selector  InputPortWidth=4  IndexOptions=Index vector (dialog)  Indices=[4]  OutputSizes=1
  Selector1 : Selector  InputPortWidth=3  IndexOptions=Index vector (dialog)  Indices=[3]  OutputSizes=1
  Selector2 : Selector  InputPortWidth=3  IndexOptions=Index vector (dialog)  Indices=[1 2]  OutputSizes=1
  Selector3 : Selector  InputPortWidth=3  IndexOptions=Index vector (dialog)  Indices=[1 2]  OutputSizes=1
  Terminator : Terminator
  Status : Outport
  AACSP : Outport  Port=2
  wires:
  Constant3/1 -> Bus Creator/4  "L1"
  Data Type Conversion/1 -> Status/1
  Bus Creator/1 -> AACSP/1
  ToWP/1 -> Bus Selector2/1, Bus Selector3/1
  Constant1/1 -> Bus Creator/5  "climbrate"
  Bus Selector3/1 -> Selector/1  "<params>"
  Selector/1 -> Bus Creator/1  "airspeed"
  States/1 -> Bus Selector4/1
  Bus Selector4/1 -> Selector3/1, Selector1/1  "<Xe>"
  Selector1/1 -> Gain/1
  Gain/1 -> Bus Creator/2  "alt"
  Constant4/1 -> Bus Creator/3  "course"
  Constant5/1 -> Data Type Conversion/1
  Bus Selector2/1 -> Selector2/1  "<position>"
  FromWP/1 -> Terminator/1

== system VTOLAutopilotController/Guidance Test Bench/ControlType/Guidance Testbench/Guidance Logic/Guidance Stateflow/Guidance Mode Selector/GuidanceLogic.FixedWingEntry.FixedWingStabilize.Stabilize ==
  States : Inport
  Action Port : ActionPort
      settings: CopyFcn=Stateflow.SLINSF.SimulinkMan.removeBlockPreDeleteFcn  PreDeleteFcn=Stateflow.SLINSF.SimulinkMan.unsafePredeleteFcn
  1-D Lookup Table : Lookup_n-D  NumberOfTableDimensions=1  BreakpointsForDimension1=[controlParams.VtransitionFWD1 controlParams.VtransitionFWD2]  Table=[0 controlParams.PitchtransitionFWD]  ExtrapMethod=Clip  InternalRulePriority=Speed  RndMeth=Simplest
  Bus Creator2 : BusCreator  Inputs=5  OutDataTypeStr=Bus: FixedWingCommandBus  NonVirtualBus=on
      settings: InheritFromInputs=off
  Bus Selector1 : BusSelector  OutputSignals=Ve
  Bus Selector2 : BusSelector  OutputSignals=Euler
  Constant{,1,4,6} (4 alike) : Constant  Value=0
  Constant7 : Constant  Value=65*const.kts2mps
  Data Type Conversion : DataTypeConversion  OutDataTypeStr=uint8  SaturateOnIntegerOverflow=off  RndMeth=Floor
  Forward velocity : Subsystem
  Selector3 : Selector  InputPortWidth=3  IndexOptions=Index vector (dialog)  Indices=[3]  OutputSizes=1
  Selector4 : Selector  InputPortWidth=3  IndexOptions=Index vector (dialog)  Indices=[2]  OutputSizes=1
  Selector5 : Selector  InputPortWidth=3  IndexOptions=Index vector (dialog)  Indices=[1]  OutputSizes=1
  SinCos1 : Trigonometry  Operator=sincos
  Status : Outport
  FixedWingSP : Outport  Port=2
  wires:
  Data Type Conversion/1 -> Status/1
  Constant/1 -> Data Type Conversion/1
  States/1 -> Bus Selector2/1, Bus Selector1/1
  Bus Creator2/1 -> FixedWingSP/1
  Constant4/1 -> Bus Creator2/1  "roll"
  Constant6/1 -> Bus Creator2/3  "yaw"
  Constant7/1 -> Bus Creator2/4  "airspeed"
  Selector5/1 -> Forward velocity/2(vx)
  Forward velocity/1(ef) -> 1-D Lookup Table/1  "vf"
  SinCos1/1 -> Forward velocity/3(sin)
  Bus Selector2/1 -> Selector3/1  "<Euler>"
  Selector4/1 -> Forward velocity/1(vy)
  Bus Selector1/1 -> Selector5/1, Selector4/1  "<Ve>"
  SinCos1/2 -> Forward velocity/4(cos)
  Selector3/1 -> SinCos1/1  "yaw"
  1-D Lookup Table/1 -> Bus Creator2/2  "pitch"
  Constant1/1 -> Bus Creator2/5  "flap"

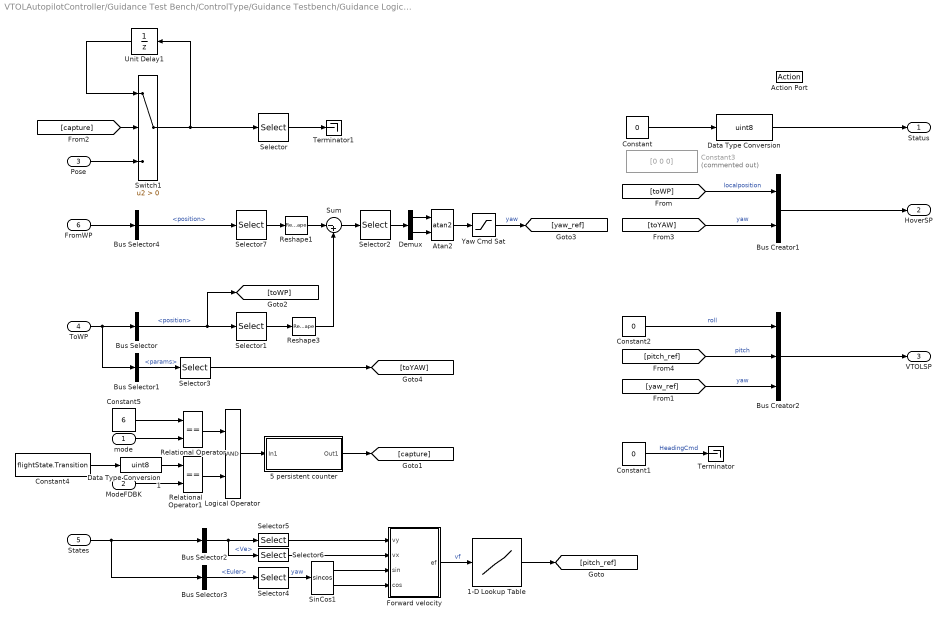
== system VTOLAutopilotController/Guidance Test Bench/ControlType/Guidance Testbench/Guidance Logic/Guidance Stateflow/Guidance Mode Selector/GuidanceLogic.ForwardTransitionBegin ==
  mode : Inport
  ModeFDBK : Inport  Port=2
  Pose : Inport  Port=3
  ToWP : Inport  Port=4
  States : Inport  Port=5
  FromWP : Inport  Port=6
  Action Port : ActionPort
      settings: CopyFcn=Stateflow.SLINSF.SimulinkMan.removeBlockPreDeleteFcn  PreDeleteFcn=Stateflow.SLINSF.SimulinkMan.unsafePredeleteFcn
  1-D Lookup Table : Lookup_n-D  NumberOfTableDimensions=1  BreakpointsForDimension1=[controlParams.VtransitionFWD1 controlParams.VtransitionFWD2]  Table=[0 controlParams.PitchtransitionFWD]  ExtrapMethod=Clip  InternalRulePriority=Speed  RndMeth=Simplest
  5 persistent counter : Subsystem
  Atan2 : Trigonometry  Operator=atan2
  Bus Creator1 : BusCreator  Inputs=2  OutDataTypeStr=Bus: LAPY  NonVirtualBus=on
  Bus Creator2 : BusCreator  Inputs=3  OutDataTypeStr=Bus: VTOLCommandBus  NonVirtualBus=on
  Bus Selector : BusSelector  OutputSignals=position
  Bus Selector1 : BusSelector  OutputSignals=params
  Bus Selector2 : BusSelector  OutputSignals=Ve
  Bus Selector3 : BusSelector  OutputSignals=Euler
  Bus Selector4 : BusSelector  OutputSignals=position
  Constant : Constant  Value=0
  Constant1 : Constant  Value=0
  Constant2 : Constant  Value=0
  Constant3 : Constant  Commented=on  Value=[0 0 0]
  Constant4 : Constant  Value=flightState.Transition
  Constant5 : Constant  Value=6
  Data Type Conversion : DataTypeConversion  OutDataTypeStr=uint8  SaturateOnIntegerOverflow=off  RndMeth=Floor
  Data Type Conversion1 : DataTypeConversion  OutDataTypeStr=uint8  SaturateOnIntegerOverflow=off  RndMeth=Floor
  Demux : Demux  Outputs=2
  Forward velocity : Subsystem
  Logical Operator : Logic  AllPortsSameDT=off  OutDataTypeStr=boolean
  Relational Operator : RelationalOperator  Operator===  OutDataTypeStr=boolean  RndMeth=Simplest  InputSameDT=off
  Relational Operator1 : RelationalOperator  Operator===  OutDataTypeStr=boolean  RndMeth=Simplest  InputSameDT=off
  Reshape1 : Reshape
  Reshape3 : Reshape
  Selector : Selector  InputPortWidth=4  IndexOptions=Index vector (dialog)  Indices=[1 2]  OutputSizes=1
  Selector1 : Selector  InputPortWidth=3  IndexOptions=Index vector (dialog)  Indices=[1 2]  OutputSizes=1
  Selector2 : Selector  InputPortWidth=2  IndexOptions=Index vector (dialog)  Indices=[2 1]  OutputSizes=1
  Selector3 : Selector  InputPortWidth=4  IndexOptions=Index vector (dialog)  Indices=[1]  OutputSizes=1
  Selector4 : Selector  InputPortWidth=3  IndexOptions=Index vector (dialog)  Indices=[3]  OutputSizes=1
  Selector5 : Selector  InputPortWidth=3  IndexOptions=Index vector (dialog)  Indices=[2]  OutputSizes=1
  Selector6 : Selector  InputPortWidth=3  IndexOptions=Index vector (dialog)  Indices=[1]  OutputSizes=1
  Selector7 : Selector  InputPortWidth=3  IndexOptions=Index vector (dialog)  Indices=[1 2]  OutputSizes=1
  SinCos1 : Trigonometry  Operator=sincos
  Sum : Sum  Inputs=|-+
  Switch1 : Switch  Criteria=u2 > Threshold  SaturateOnIntegerOverflow=off  InputSameDT=off
  Terminator : Terminator
  Terminator1 : Terminator
  Unit Delay1 : UnitDelay  InitialCondition=zeros(4,1)  SampleTime=-1  HasFrameUpgradeWarning=on
  Yaw Cmd Sat : Saturate  UpperLimit=pi  LowerLimit=-pi
      settings: AttributesFormatString=[%<UpperLimit> %<LowerLimit>]
  Status : Outport
  HoverSP : Outport  Port=2
  VTOLSP : Outport  Port=3
  wires:
  Bus Creator1/1 -> HoverSP/1
  Data Type Conversion/1 -> Status/1
  Constant/1 -> Data Type Conversion/1
  Constant1/1 -> Terminator/1  "HeadingCmd"
  5 persistent counter/1(Out1) -> [capture]
  ModeFDBK/1 -> Relational Operator1/2
  Logical Operator/1 -> 5 persistent counter/1(In1)
  Relational Operator/1 -> Logical Operator/1
  Constant4/1 -> Data Type Conversion1/1
  Relational Operator1/1 -> Logical Operator/2
  mode/1 -> Relational Operator/2
  Constant5/1 -> Relational Operator/1
  Data Type Conversion1/1 -> Relational Operator1/1
  Switch1/1 -> Selector/1, Unit Delay1/1
  Unit Delay1/1 -> Switch1/1
  [capture] -> Switch1/2
  Pose/1 -> Switch1/3
  Selector1/1 -> Reshape3/1
  Bus Selector/1 -> [toWP], Selector1/1  "<position>"
  Selector2/1 -> Demux/1
  Demux/1 -> Atan2/1
  Demux/2 -> Atan2/2
  Atan2/1 -> Yaw Cmd Sat/1
  Reshape3/1 -> Sum/2
  Sum/1 -> Selector2/1
  Bus Creator2/1 -> VTOLSP/1
  ToWP/1 -> Bus Selector1/1, Bus Selector/1
  Yaw Cmd Sat/1 -> [yaw_ref]  "yaw"
  [yaw_ref] -> Bus Creator2/3  "yaw"
  Constant2/1 -> Bus Creator2/1  "roll"
  [pitch_ref] -> Bus Creator2/2  "pitch"
  Bus Selector1/1 -> Selector3/1  "<params>"
  Selector3/1 -> [toYAW]
  [toYAW] -> Bus Creator1/2  "yaw"
  [toWP] -> Bus Creator1/1  "localposition"
  SinCos1/1 -> Forward velocity/3(sin)
  Bus Selector3/1 -> Selector4/1  "<Euler>"
  Selector4/1 -> SinCos1/1  "yaw"
  States/1 -> Bus Selector3/1, Bus Selector2/1
  Bus Selector2/1 -> Selector6/1, Selector5/1  "<Ve>"
  SinCos1/2 -> Forward velocity/4(cos)
  Selector6/1 -> Forward velocity/2(vx)
  Selector5/1 -> Forward velocity/1(vy)
  Forward velocity/1(ef) -> 1-D Lookup Table/1  "vf"
  1-D Lookup Table/1 -> [pitch_ref]
  FromWP/1 -> Bus Selector4/1
  Selector7/1 -> Reshape1/1
  Reshape1/1 -> Sum/1
  Bus Selector4/1 -> Selector7/1  "<position>"
  Selector/1 -> Terminator1/1

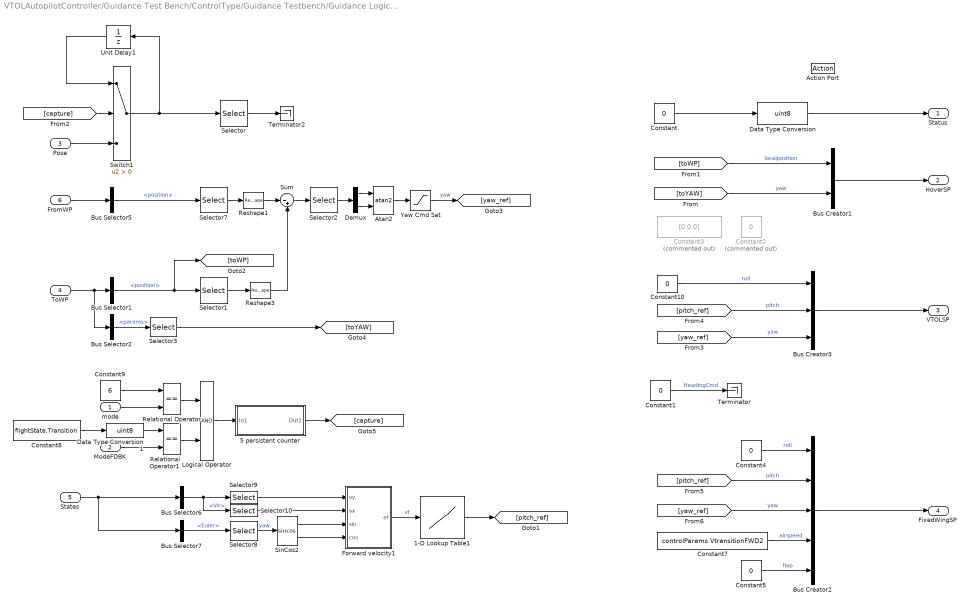
== system VTOLAutopilotController/Guidance Test Bench/ControlType/Guidance Testbench/Guidance Logic/Guidance Stateflow/Guidance Mode Selector/GuidanceLogic.ForwardTransitionIntermediate ==
  mode : Inport
  ModeFDBK : Inport  Port=2
  Pose : Inport  Port=3
  ToWP : Inport  Port=4
  States : Inport  Port=5
  FromWP : Inport  Port=6
  Action Port : ActionPort
      settings: CopyFcn=Stateflow.SLINSF.SimulinkMan.removeBlockPreDeleteFcn  PreDeleteFcn=Stateflow.SLINSF.SimulinkMan.unsafePredeleteFcn
  1-D Lookup Table1 : Lookup_n-D  NumberOfTableDimensions=1  BreakpointsForDimension1=[controlParams.VtransitionFWD1 controlParams.VtransitionFWD2]  Table=[0 controlParams.PitchtransitionFWD]  ExtrapMethod=Clip  InternalRulePriority=Speed  RndMeth=Simplest
  5 persistent counter : Subsystem
  Atan2 : Trigonometry  Operator=atan2
  Bus Creator1 : BusCreator  Inputs=2  OutDataTypeStr=Bus: LAPY  NonVirtualBus=on
      settings: InheritFromInputs=off
  Bus Creator2 : BusCreator  Inputs=5  OutDataTypeStr=Bus: FixedWingCommandBus  NonVirtualBus=on
      settings: InheritFromInputs=off
  Bus Creator3 : BusCreator  Inputs=3  OutDataTypeStr=Bus: VTOLCommandBus  NonVirtualBus=on
  Bus Selector1 : BusSelector  OutputSignals=position
  Bus Selector2 : BusSelector  OutputSignals=params
  Bus Selector5 : BusSelector  OutputSignals=position
  Bus Selector6 : BusSelector  OutputSignals=Ve
  Bus Selector7 : BusSelector  OutputSignals=Euler
  Constant{,1,4..5,10} (5 alike) : Constant  Value=0
  Constant2 : Constant  Commented=on  Value=0
  Constant3 : Constant  Commented=on  Value=[0 0 0]
  Constant7 : Constant  Value=controlParams.VtransitionFWD2
  Constant8 : Constant  Value=flightState.Transition
  Constant9 : Constant  Value=6
  Data Type Conversion : DataTypeConversion  OutDataTypeStr=uint8  SaturateOnIntegerOverflow=off  RndMeth=Floor
  Data Type Conversion1 : DataTypeConversion  OutDataTypeStr=uint8  SaturateOnIntegerOverflow=off  RndMeth=Floor
  Demux : Demux  Outputs=2
  Forward velocity1 : Subsystem
  Logical Operator : Logic  AllPortsSameDT=off  OutDataTypeStr=boolean
  Relational Operator : RelationalOperator  Operator===  OutDataTypeStr=boolean  RndMeth=Simplest  InputSameDT=off
  Relational Operator1 : RelationalOperator  Operator===  OutDataTypeStr=boolean  RndMeth=Simplest  InputSameDT=off
  Reshape1 : Reshape
  Reshape3 : Reshape
  Selector : Selector  InputPortWidth=4  IndexOptions=Index vector (dialog)  Indices=[1 2]  OutputSizes=1
  Selector1 : Selector  InputPortWidth=3  IndexOptions=Index vector (dialog)  Indices=[1 2]  OutputSizes=1
  Selector10 : Selector  InputPortWidth=3  IndexOptions=Index vector (dialog)  Indices=[1]  OutputSizes=1
  Selector2 : Selector  InputPortWidth=2  IndexOptions=Index vector (dialog)  Indices=[2 1]  OutputSizes=1
  Selector3 : Selector  InputPortWidth=4  IndexOptions=Index vector (dialog)  Indices=[1]  OutputSizes=1
  Selector7 : Selector  InputPortWidth=3  IndexOptions=Index vector (dialog)  Indices=[1 2]  OutputSizes=1
  Selector8 : Selector  InputPortWidth=3  IndexOptions=Index vector (dialog)  Indices=[3]  OutputSizes=1
  Selector9 : Selector  InputPortWidth=3  IndexOptions=Index vector (dialog)  Indices=[2]  OutputSizes=1
  SinCos2 : Trigonometry  Operator=sincos
  Sum : Sum  Inputs=|-+
  Switch1 : Switch  Criteria=u2 > Threshold  SaturateOnIntegerOverflow=off  InputSameDT=off
  Terminator : Terminator
  Terminator2 : Terminator
  Unit Delay1 : UnitDelay  InitialCondition=zeros(4,1)  SampleTime=-1  HasFrameUpgradeWarning=on
  Yaw Cmd Sat : Saturate  UpperLimit=pi  LowerLimit=-pi
      settings: AttributesFormatString=[%<UpperLimit> %<LowerLimit>]
  Status : Outport
  HoverSP : Outport  Port=2
  VTOLSP : Outport  Port=3
  FixedWingSP : Outport  Port=4
  wires:
  Bus Creator1/1 -> HoverSP/1
  Data Type Conversion/1 -> Status/1
  Constant/1 -> Data Type Conversion/1
  Constant1/1 -> Terminator/1  "HeadingCmd"
  Bus Creator2/1 -> FixedWingSP/1
  Constant4/1 -> Bus Creator2/1  "roll"
  [pitch_ref] -> Bus Creator2/2  "pitch"
  [yaw_ref] -> Bus Creator2/3  "yaw"
  Constant7/1 -> Bus Creator2/4  "airspeed"
  Reshape3/1 -> Sum/2
  Demux/2 -> Atan2/2
  Selector/1 -> Terminator2/1
  Selector2/1 -> Demux/1
  Selector3/1 -> [toYAW]
  Sum/1 -> Selector2/1
  Pose/1 -> Switch1/3
  Demux/1 -> Atan2/1
  Bus Selector2/1 -> Selector3/1  "<params>"
  Reshape1/1 -> Sum/1
  FromWP/1 -> Bus Selector5/1
  Selector1/1 -> Reshape3/1
  Unit Delay1/1 -> Switch1/1
  [capture] -> Switch1/2
  Atan2/1 -> Yaw Cmd Sat/1
  Bus Selector5/1 -> Selector7/1  "<position>"
  Selector7/1 -> Reshape1/1
  Bus Selector1/1 -> [toWP], Selector1/1  "<position>"
  Switch1/1 -> Selector/1, Unit Delay1/1
  Yaw Cmd Sat/1 -> [yaw_ref]  "yaw"
  ToWP/1 -> Bus Selector2/1, Bus Selector1/1
  States/1 -> Bus Selector7/1, Bus Selector6/1
  Constant8/1 -> Data Type Conversion1/1
  Data Type Conversion1/1 -> Relational Operator1/1
  ModeFDBK/1 -> Relational Operator1/2
  5 persistent counter/1(Out1) -> [capture]
  Relational Operator/1 -> Logical Operator/1
  Logical Operator/1 -> 5 persistent counter/1(In1)
  Selector9/1 -> Forward velocity1/1(vy)
  mode/1 -> Relational Operator/2
  Bus Selector6/1 -> Selector10/1, Selector9/1  "<Ve>"
  Relational Operator1/1 -> Logical Operator/2
  Selector8/1 -> SinCos2/1  "yaw"
  Selector10/1 -> Forward velocity1/2(vx)
  SinCos2/1 -> Forward velocity1/3(sin)
  Forward velocity1/1(ef) -> 1-D Lookup Table1/1  "vf"
  Constant9/1 -> Relational Operator/1
  1-D Lookup Table1/1 -> [pitch_ref]
  SinCos2/2 -> Forward velocity1/4(cos)
  Bus Selector7/1 -> Selector8/1  "<Euler>"
  [toYAW] -> Bus Creator1/2  "yaw"
  [toWP] -> Bus Creator1/1  "localposition"
  Constant10/1 -> Bus Creator3/1  "roll"
  [pitch_ref] -> Bus Creator3/2  "pitch"
  Bus Creator3/1 -> VTOLSP/1
  [yaw_ref] -> Bus Creator3/3  "yaw"
  Constant5/1 -> Bus Creator2/5  "flap"
